simulink model "FilteredX_LMS_ANC"  (R2022a)
settings: Solver=FixedStepDiscrete  StartTime=0.0  StopTime=10  RelTol=1e-3
libraries: dspadpt3 x1, dspsrcs4 x1
settings Model: Creator=The MathWorks, Inc.  LastModifiedBy=The MathWorks, Inc.
settings SolverCC: AlgebraicLoopSolver=TrustRegion
settings DataIOCC: ReturnWorkspaceOutputs=off
settings DebuggingCC: UnconnectedInputMsg=warning  UnconnectedOutputMsg=warning  UnconnectedLineMsg=warning  SFMachineParentedDataDiag=warning  ArithmeticOperatorsInVariantConditions=warning
settings SFSimCC: CustomCodeUndefinedFunction=UseInterfaceOnly

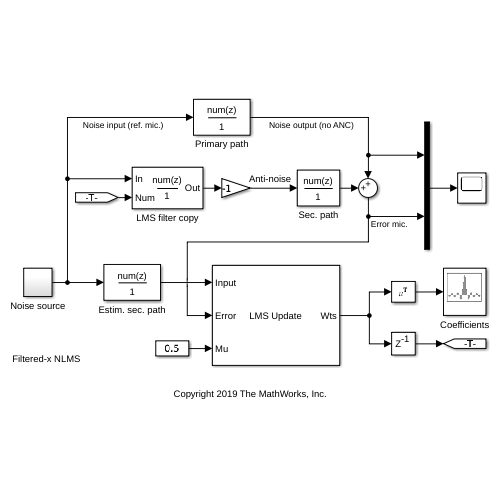
[thumbnail: Simulink's stored preview of the top-level diagram]
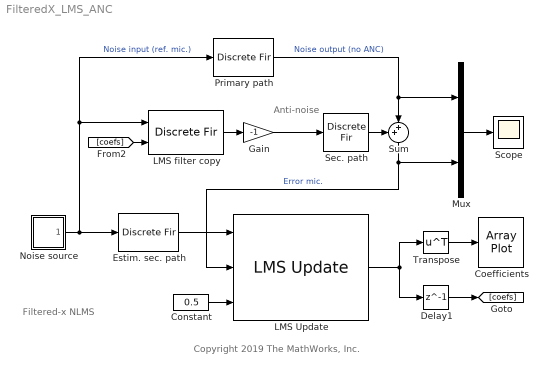
== system FilteredX_LMS_ANC ==
  note: Filtered-x NLMS
  note: Anti-noise
  note: Copyright 2019 The MathWorks, Inc.
  Coefficients : ArrayPlot  WindowPosition=[1954.000000,667.000000,800.000000,412.000000,]  Visible=on  ScopeFrameLocation=window  AxesScaling=Manual  YLimits=[-0.373494,0.373651]  DefaultConfigurationName=dsp.scopes.ArrayPlotBlockSpecification
  Constant : Constant  Value=0.5
  Delay1 : Delay  DelayLength=1
  Estim. sec. path : DiscreteFir  Coefficients="[0.466  0.533  -0.257  -0.274  -0.231  -0.175]"
  Gain : Gain  Gain=-1
  LMS Update : dspadpt3/LMS Update  Method=Normalized LMS  Length=24  NumFilters=1  StepSizeSource=Input port  StepSize=0.1  LeakageFactor=1.0  InitialConditions=0  AdaptiveFilterMode=Tapped delay-line FIR filter  EnableAdaptInput=off  EnableResetInput=off  SimulateUsing=Interpreted execution
      settings: SourceProductBaseCode=DS
  LMS filter copy : DiscreteFir  CoefSource=Input port
      settings: InputPortMap=u0,u1
  Mux : Mux  Inputs=2
  Noise source : Subsystem
  Primary path : DiscreteFir  Coefficients=conv([0.5 0.5 -.3 -.3 -.2 -.2],[.1 -.1 .2 -.2 .3 -.3 .15 -.15])
  Scope : Scope
  Sec. path : DiscreteFir  Coefficients=[0.5 0.5 -.3 -.3 -.2 -.2]
  Sum : Sum  Inputs=++|
  Transpose : Math  Operator=transpose  SignedPower=on
  wires:
  Primary path/1 -> Mux/1, Sum/2  "Noise output (no ANC)"
  LMS filter copy/1 -> Gain/1
  Sum/1 -> LMS Update/2, Mux/2  "Error mic."
  Sec. path/1 -> Sum/1
  Estim. sec. path/1 -> LMS Update/1
  Mux/1 -> Scope/1
  LMS Update/1 -> Transpose/1, Delay1/1
  [coefs] -> LMS filter copy/2
  Noise source/1(Out1) -> Estim. sec. path/1, LMS filter copy/1, Primary path/1  "Noise input (ref. mic.)"
  Constant/1 -> LMS Update/3
  Transpose/1 -> Coefficients/1
  Delay1/1 -> [coefs]
  Gain/1 -> Sec. path/1

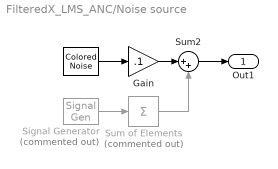
== system FilteredX_LMS_ANC/Noise source ==
  " " : dspsrcs4/Colored Noise  Color=white  InverseFrequencyPower=1  BoundedOutput=off  NumChannels=1  OutputDataType=double  SamplesPerFrame=1  SampleTime=1/8000  RandomStream=mt19937ar with seed  Seed=67  SimulateUsing=Interpreted execution
      settings: SourceProductBaseCode=DS
  Gain : Gain  Gain=.1
  Signal Generator : SignalGenerator  Commented=on  Frequency=[150 250 350]
  Sum of Elements : Sum  Commented=on  Inputs=+
  Sum2 : Sum  Inputs=|++
  Out1 : Outport  VectorParamsAs1DForOutWhenUnconnected=off
  wires:
  Signal Generator/1 -> Sum of Elements/1
  Gain/1 -> Sum2/1
  Sum of Elements/1 -> Sum2/2
  " "/1 -> Gain/1
  Sum2/1 -> Out1/1
